simulink model "Lab5"  (R2024b)
settings: Solver=VariableStepAuto  StartTime=0.0  StopTime=inf  RelTol=1e-3
undefined symbols (not defined in the file): EbNo
libraries: commdigbbndpm3 x2, commblkcod2 x2, commchan3 x1, commrandsrc3 x1, commsink2 x1
settings Model: Creator=Jose  LastModifiedBy=Jose

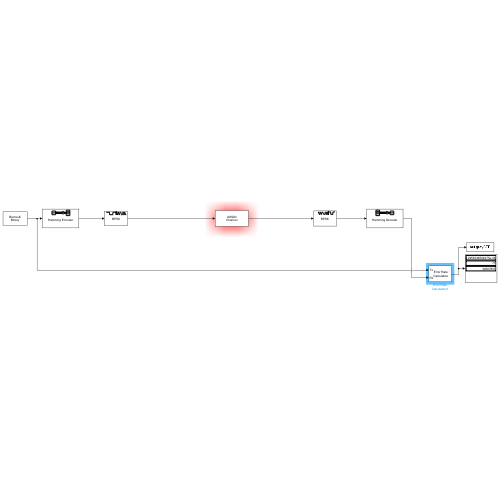
[thumbnail: Simulink's stored preview of the top-level diagram]
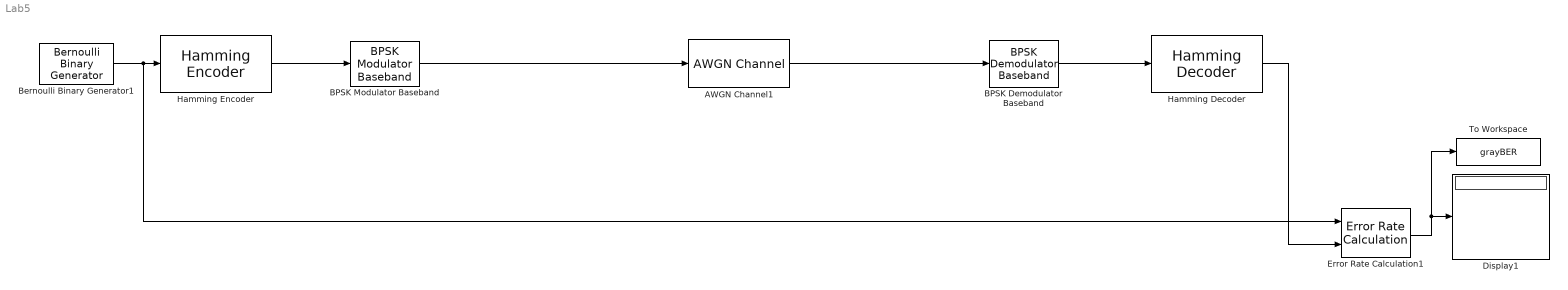
== system Lab5 ==
  AWGN Channel1 : commchan3/AWGN Channel  LegacyMode=off  NoiseMethod="Signal to noise ratio  (Eb/No)"  noiseMode="Signal to noise ratio  (SNR)"  EbNo=EbNo + 10*log10(11/15)  EsNo=10  SNR=10  BitsPerSymbol=1  SignalPower=1  SamplesPerSymbol=1  SymbolPeriod=1  VarianceSource=Parameter  Variance=1  RandomStream=mt19937ar with seed  Seed=67  SimulateUsing=Code generation
  BPSK Demodulator Baseband : commdigbbndpm3/BPSK Demodulator Baseband  DecType=Hard decision  VarSource=Dialog  Variance=0.5  Ph=0  outDtype=double  derotateFactorWordLen=16  derotateFactorDataTypeStr=Inherit: Same word length as input  derotateFactorLastDataTypeStr=Inherit: Same word length as input
      settings: LibrarySourceBlock=|
      | commhdldigbbndpm/BPSK
      | Demodulator
      | Baseband
  BPSK Modulator Baseband : commdigbbndpm3/BPSK Modulator Baseband  Ph=0  outDtype=double  outWordLen=16  outUDDataType=sfix(16)  outFracLenMode=Best precision  outFracLen=15  outDataTypeStr=double  outLastDataTypeStr=double
      settings: LibrarySourceBlock=|
      | commhdldigbbndpm/BPSK
      | Modulator
      | Baseband
  Bernoulli Binary Generator1 : commrandsrc3/Bernoulli Binary Generator  ProbabilityOfZero=0.5  SeedSource=Auto  Seed=67  SampleTime=1e-6  SamplesPerFrame=11  OutputDataType=double  SimulateUsing=Interpreted execution
  Display1 : Display
  Error Rate Calculation1 : commsink2/Error Rate Calculation  N=0  st_delay=0  cp_mode=Entire frame  subframe=[]  PMode=Port  WsName=ErrorVec  RsMode2=off  stop=on  numErr=100  maxBits=1e8
      settings: LibrarySourceBlock=|
      | commhdlsink/Error Rate
      | Calculation
  Hamming Decoder : commblkcod2/Hamming Decoder  n=15  k=11
  Hamming Encoder : commblkcod2/Hamming Encoder  n=15  k=11
  To Workspace : ToWorkspace  VariableName=grayBER  SampleTime=-1
      settings: MaxDataPoints=2  Save2DSignal=2-D array (concatenate along first dimension)
  wires:
  Error Rate Calculation1/1 -> To Workspace/1, Display1/1
  BPSK Modulator Baseband/1 -> AWGN Channel1/1
  Bernoulli Binary Generator1/1 -> Error Rate Calculation1/1, Hamming Encoder/1
  Hamming Encoder/1 -> BPSK Modulator Baseband/1
  AWGN Channel1/1 -> BPSK Demodulator Baseband/1
  BPSK Demodulator Baseband/1 -> Hamming Decoder/1
  Hamming Decoder/1 -> Error Rate Calculation1/2
